simulink model "removeNaNRefMod"  (R2016b)
settings: Solver=VariableStepAuto  StartTime=0.0  StopTime=10.0  RelTol=1e-3
settings Model: Creator=Taeke  LastModifiedBy=Taeke

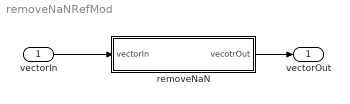
== system removeNaNRefMod ==
  vectorIn : Inport
  removeNaN : MATLAB Function  TreatAsAtomicUnit=on
  vectorOut : Outport
  wires:
  vectorIn/1 -> removeNaN/1(vectorIn)
  removeNaN/1(vecotrOut) -> vectorOut/1

== matlab function removeNaNRefMod/removeNaN ==
  data: vectorIn input; vecotrOut output [1..100]
function vecotrOut = removeNaN(vectorIn)
    vecotrOut = vectorIn(~isnan(vectorIn));
end
